simulink model "acrobot_sim_euler"  (R2013a)
settings: Solver=ode1  StartTime=0.0  StopTime=20  FixedStep=0.01  RelTol=1e-3
PreLoadFcn:
  | m1 = 1;
  | m2 = 1;
  | L1 = 1;
  | L2 = 1;
  | Lc1 = L1/2;
  | Lc2 = L2/2;
  | Ic1 = (Lc1*Lc1)/3;
  | Ic2 = (Lc2*Lc2)/3;
  | I1 = Ic1+m1*Lc1*Lc1;
  | I2 = Ic2+m2*Lc2*Lc2;
  | b1 = 0.4;
  | b2 = 0.4;
  | g = 9.8;
  | theta1_0 = -pi/8;
  | theta2_0 = 0;
StartFcn:
  | m1 = 1;
  | m2 = 1;
  | L1 = 1;
  | L2 = 1;
  | Lc1 = L1/2;
  | Lc2 = L2/2;
  | Ic1 = (Lc1*Lc1)/3;
  | Ic2 = (Lc2*Lc2)/3;
  | I1 = Ic1+m1*Lc1*Lc1;
  | I2 = Ic2+m2*Lc2*Lc2;
  | b1 = 0.4;
  | b2 = 0.4;
  | g = 9.8;
  | theta1_0 = -pi/8;
  | theta2_0 = 0;
libraries: mblibv1 x8, simulink x2
settings Model: Creator=Guy  LastModifiedBy=nightling
settings DataIOCC: SignalLoggingSaveFormat=ModelDataLogs
settings OptimizationCC: ExpressionDepthLimit=2147483647  InitFltsAndDblsToZero=on
settings DebuggingCC: AlgebraicLoopMsg=none  FcnCallInpInsideContextMsg=UseLocalSettings  StrictBusMsg=Warning
settings SFSimCC: SimParseCustomCode=off
settings GRTTargetCC: CombineOutputUpdateFcns=off  GRTInterface=on
settings SimMechanicsCC: VisOnUpdateDiagram=on  VisDuringSimulation=on  AutoFitVis=GROWTOFIT  LastVizWinPosition=[685 679 560 420]  CamPosition=[0.997125;-1.39973;13.4628;]  CamTarget=[0.997125;-1.39973;0;]  CamUpVector=[0;1;0;]  CamHeight=3.22959  VisBackgroundColor=[0.9;0.9;0.95;]  DefaultBodyColor=[1;0;0;]

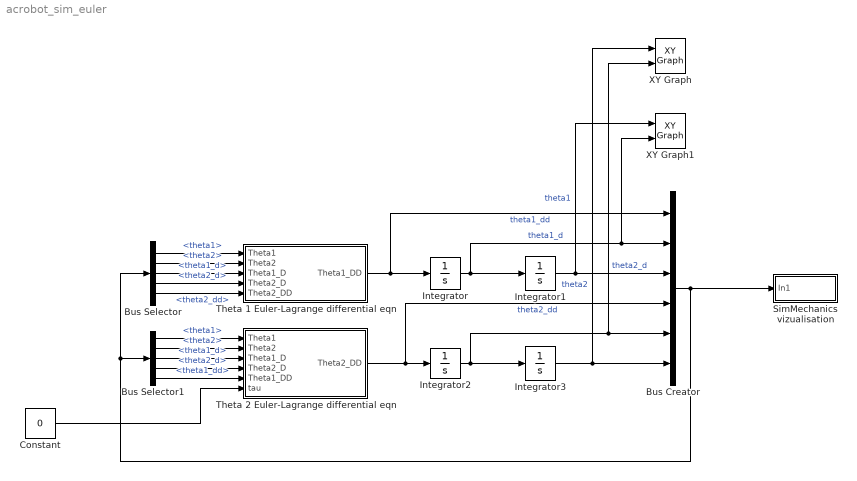
== system acrobot_sim_euler ==
  Bus Creator : BusCreator  Inputs=6
  Bus Selector : BusSelector  OutputSignals=theta1,theta2,theta1_d,theta2_d,theta2_dd
  Bus Selector1 : BusSelector  OutputSignals=theta1,theta2,theta1_d,theta2_d,theta1_dd
  Constant : Constant  Value=0
  Integrator : Integrator  InitialCondition=[0 ]
  Integrator1 : Integrator  InitialCondition=theta1_0
  Integrator2 : Integrator  InitialCondition="[0  ]"
  Integrator3 : Integrator  InitialCondition=theta2_0
  SimMechanics vizualisation : Subsystem
  Theta 1 Euler-Lagrange differential eqn : Subsystem
  Theta 2 Euler-Lagrange differential eqn : Subsystem
  XY Graph : simulink/Sinks/XY Graph  xmin=-0.5  xmax=0.5  ymin=-2  ymax=2  st=-1
  XY Graph1 : simulink/Sinks/XY Graph  xmin=-1  xmax=1  ymin=-5  ymax=5  st=-1
  wires:
  Integrator/1 -> XY Graph1/2, Bus Creator/2, Integrator1/1  "theta1_d"
  Integrator1/1 -> XY Graph1/1, Bus Creator/3  "theta1"
  Theta 1 Euler-Lagrange differential eqn/1(Theta1_DD) -> Bus Creator/1, Integrator/1  "theta1_dd"
  Theta 2 Euler-Lagrange differential eqn/1(Theta2_DD) -> Bus Creator/4, Integrator2/1  "theta2_dd"
  Integrator2/1 -> XY Graph/2, Bus Creator/5, Integrator3/1  "theta2_d"
  Integrator3/1 -> XY Graph/1, Bus Creator/6  "theta2"
  Bus Selector/1 -> Theta 1 Euler-Lagrange differential eqn/1(Theta1)  "<theta1>"
  Bus Selector/2 -> Theta 1 Euler-Lagrange differential eqn/2(Theta2)  "<theta2>"
  Bus Selector/5 -> Theta 1 Euler-Lagrange differential eqn/5(Theta2_DD)  "<theta2_dd>"
  Bus Selector/4 -> Theta 1 Euler-Lagrange differential eqn/4(Theta2_D)  "<theta2_d>"
  Bus Selector1/1 -> Theta 2 Euler-Lagrange differential eqn/1(Theta1)  "<theta1>"
  Bus Selector1/2 -> Theta 2 Euler-Lagrange differential eqn/2(Theta2)  "<theta2>"
  Bus Selector1/5 -> Theta 2 Euler-Lagrange differential eqn/5(Theta1_DD)  "<theta1_dd>"
  Bus Selector1/3 -> Theta 2 Euler-Lagrange differential eqn/3(Theta1_D)  "<theta1_d>"
  Bus Selector/3 -> Theta 1 Euler-Lagrange differential eqn/3(Theta1_D)  "<theta1_d>"
  Bus Selector1/4 -> Theta 2 Euler-Lagrange differential eqn/4(Theta2_D)  "<theta2_d>"
  Bus Creator/1 -> Bus Selector/1, Bus Selector1/1, SimMechanics vizualisation/1(In1)
  Constant/1 -> Theta 2 Euler-Lagrange differential eqn/6(tau)

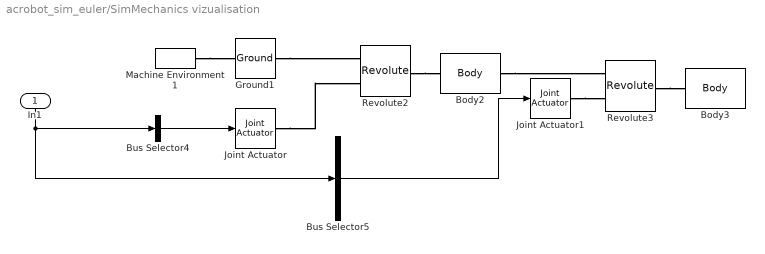
== system acrobot_sim_euler/SimMechanics vizualisation ==
  In1 : Inport
  Body2 : mblibv1/Bodies/Body  LConnTagsString=CS1  RConnTagsString=CS2  UpdateFromCAD=off  DialogClass=MechanicalBodyBlock  Mass=m1  MassUnits=kg  InertiaUnits=kg*m^2  Inertia=zeros(3)  Shape=Cylinder  ShapeDims=[1 1]  ShapeUnits=m  ShapeUse=false  Density=1  DensityUnits=kg/m^3  DensityUse=false  GraphicsMode=MACHINE_DEFAULT  BodyColorSelMode=COLORPALETTE  BodyColor=[0.043137 0.51765 0.78039]  AttachedToCS=CG  CG=Left$CG$[0 -L1/2 0]$CS1$CS1$m$[0 0 0]$Euler X-Y-Z$deg$WORLD$false$none  WorkingFrames=Left$CS1$[0 0 0]$Adjoining$Adjoining$m$[0 0 0]$Euler X-Y-Z$deg$WORLD$true$none#Right$CS2$[0 -L1 0]$CS1$CS1$m$[0 0 0]$Euler X-Y-Z$deg$WORLD$true$none  CGPos=[0 -L1/2 0]  CGRot=[0 0 0]  CS0Pos=[]  CS0Rot=[]  CS1Pos=[0 0 0]  CS1Rot=[0 0 0]  CS2Pos=[0 -L1 0]  CS2Rot=[0 0 0]  CS3Pos=[]  CS3Rot=[]  CS4Pos=[]  CS4Rot=[]  CS5Pos=[]  CS5Rot=[]  CS6Pos=[]  CS6Rot=[]  CS7Pos=[]  CS7Rot=[]  CS8Pos=[]  CS8Rot=[]  CS9Pos=[]  CS9Rot=[]  CS10Pos=[]  CS10Rot=[]  CS11Pos=[]  CS11Rot=[]  CS12Pos=[]  CS12Rot=[]  CS13Pos=[]  CS13Rot=[]  CS14Pos=[]  CS14Rot=[]  CS15Pos=[]  CS15Rot=[]  CS16Pos=[]  CS16Rot=[]  CS17Pos=[]  CS17Rot=[]  CS18Pos=[]  CS18Rot=[]  CS19Pos=[]  CS19Rot=[]  CS20Pos=[]  CS20Rot=[]
  Body3 : mblibv1/Bodies/Body  LConnTagsString=CS1  UpdateFromCAD=off  DialogClass=MechanicalBodyBlock  Mass=m2  MassUnits=kg  InertiaUnits=kg*m^2  Inertia=zeros(3)  Shape=Cylinder  ShapeDims=[1 1]  ShapeUnits=m  ShapeUse=false  Density=1  DensityUnits=kg/m^3  DensityUse=false  GraphicsMode=MACHINE_DEFAULT  BodyColorSelMode=COLORPALETTE  BodyColor=[0.043137 0.51765 0.78039]  AttachedToCS=CG  CG=Left$CG$[0 -L2/2 0]$CS1$CS1$m$[0 0 0]$Euler X-Y-Z$deg$WORLD$false$none  WorkingFrames=Left$CS1$[0 0 0]$Adjoining$Adjoining$m$[0 0 0]$Euler X-Y-Z$deg$WORLD$true$none#Right$CS2$[0 -L2 0]$CS1$CS1$m$[0 0 0]$Euler X-Y-Z$deg$WORLD$false$none  CGPos=[0 -L2/2 0]  CGRot=[0 0 0]  CS0Pos=[]  CS0Rot=[]  CS1Pos=[0 0 0]  CS1Rot=[0 0 0]  CS2Pos=[0 -L2 0]  CS2Rot=[0 0 0]  CS3Pos=[]  CS3Rot=[]  CS4Pos=[]  CS4Rot=[]  CS5Pos=[]  CS5Rot=[]  CS6Pos=[]  CS6Rot=[]  CS7Pos=[]  CS7Rot=[]  CS8Pos=[]  CS8Rot=[]  CS9Pos=[]  CS9Rot=[]  CS10Pos=[]  CS10Rot=[]  CS11Pos=[]  CS11Rot=[]  CS12Pos=[]  CS12Rot=[]  CS13Pos=[]  CS13Rot=[]  CS14Pos=[]  CS14Rot=[]  CS15Pos=[]  CS15Rot=[]  CS16Pos=[]  CS16Rot=[]  CS17Pos=[]  CS17Rot=[]  CS18Pos=[]  CS18Rot=[]  CS19Pos=[]  CS19Rot=[]  CS20Pos=[]  CS20Rot=[]
  Bus Selector4 : BusSelector  OutputSignals=theta1,theta1_d,theta1_dd  OutputAsBus=on
  Bus Selector5 : BusSelector  OutputSignals=theta2,theta2_d,theta2_dd  OutputAsBus=on
  Ground1 : mblibv1/Bodies/Ground  UpdateFromCAD=off  LeftPortType=env  RightPortType=workingframe  PhysicalDomain=Mechanical  DialogClass=GroundBlock  CoordPosition=[1 0 0]  CoordPositionUnits=m  StateVectorMgrId=1  MachineId=[2 0]  ShowEnvPort=on
  Joint Actuator : mblibv1/Sensors &  Actuators/Joint Actuator  UpdateFromCAD=off  PhysicalDomain=Mechanical  PortType=blob  ActuationStyle=Motion  AngleUnits=rad  ArcVelocityUnits=rad/s  ArcAccelerationUnits=rad/s^2  CoordPositionUnits=m  VelocityUnits=m/s  AccelerationUnits=m/s^2  ForceUnits=N  TorqueUnits=N*m  ActiveIO=on  Width=3  DialogClass=MechanicalActuatorBlock  Primitive=R1  ReferenceFrame=Absolute (World)
  Joint Actuator1 : mblibv1/Sensors &  Actuators/Joint Actuator  UpdateFromCAD=off  PhysicalDomain=Mechanical  PortType=blob  ActuationStyle=Motion  AngleUnits=rad  ArcVelocityUnits=rad/s  ArcAccelerationUnits=rad/s^2  CoordPositionUnits=m  VelocityUnits=m/s  AccelerationUnits=m/s^2  ForceUnits=N  TorqueUnits=N*m  ActiveIO=on  Width=3  DialogClass=MechanicalActuatorBlock  Primitive=R1  ReferenceFrame=Absolute (World)
  Machine Environment1 : mblibv1/Bodies/Machine Environment  PortType=env  PhysicalDomain=Mechanical  DialogTemplateClass=MECH.MachineEnvironment  SyncWhenCopied=off  Gravity=[0 -9.81 0]  GravityUnits=m/s^2  GravityAsSignal=off  Dimensionality=Auto-detect  AnalysisType=Forward dynamics  LinearAssemblyTolerance=1e-3  LinearAssemblyToleranceUnits=m  AngularAssemblyTolerance=1e-3  AngularAssemblyToleranceUnits=rad  ConstraintSolverType=Stabilizing  ConstraintRelTolerance=1e-4  ConstraintAbsTolerance=1e-4  UseRobustSingularityHandling=off  RedundancyAnalysisToleranceType=Automatically select tolerance  RedundancyAnalysisTolerance=1e-14  StatePerturbationType=Fixed  PerturbationSize=1e-5  VisualizeMachine=on  BodyVisualizationType=Use model default body geometries  BodyColorSelMode=Use model default  DefaultBodyColor=[1 0 0]
  Revolute2 : mblibv1/Joints/Revolute  LConnTagsString=__newl0|SA1  RConnTagsString=__newr0  UpdateFromCAD=off  NumSAPorts=1  CutJoint=off  MarkAsCut=off  Primitives=prismatic  PrimitiveProps=R1$World$[0 0 1]$revolute  DialogClass=JointBlock  R1Axis=[0 0 1]
  Revolute3 : mblibv1/Joints/Revolute  LConnTagsString=__newl0|SA1  RConnTagsString=__newr0  UpdateFromCAD=off  NumSAPorts=1  CutJoint=off  MarkAsCut=off  Primitives=prismatic  PrimitiveProps=R1$World$[0 0 1]$revolute  DialogClass=JointBlock  R1Axis=[0 0 1]
  wires:
  Bus Selector4/1 -> Joint Actuator/1
  In1/1 -> Bus Selector5/1, Bus Selector4/1
  Bus Selector5/1 -> Joint Actuator1/1
  connections:
  Revolute2/RConn1 -- Body2/LConn1
  Body2/RConn1 -- Revolute3/LConn1
  Revolute3/RConn1 -- Body3/LConn1
  Machine Environment1/RConn1 -- Ground1/LConn1
  Ground1/RConn1 -- Revolute2/LConn1
  Joint Actuator/RConn1 -- Revolute2/LConn2
  Joint Actuator1/RConn1 -- Revolute3/LConn2

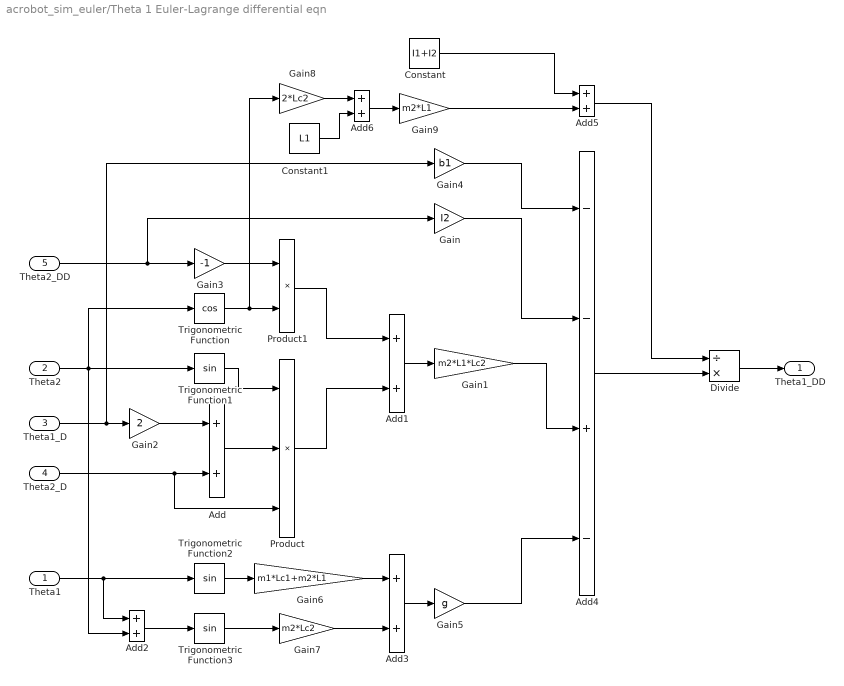
== system acrobot_sim_euler/Theta 1 Euler-Lagrange differential eqn ==
  Theta1 : Inport
  Theta2 : Inport  Port=2
  Theta1_D : Inport  Port=3
  Theta2_D : Inport  Port=4
  Theta2_DD : Inport  Port=5
  Add{,1..3,5..6} (6 alike) : Sum
  Add4 : Sum  Inputs=--+-
  Constant : Constant  Value=I1+I2
  Constant1 : Constant  Value=L1
  Divide : Product  Inputs=/*
  Gain : Gain  Gain=I2
  Gain1 : Gain  Gain=m2*L1*Lc2
  Gain2 : Gain  Gain=2
  Gain3 : Gain  Gain=-1
  Gain4 : Gain  Gain=b1
  Gain5 : Gain  Gain=g
  Gain6 : Gain  Gain=m1*Lc1+m2*L1
  Gain7 : Gain  Gain=m2*Lc2
  Gain8 : Gain  Gain=2*Lc2
  Gain9 : Gain  Gain=m2*L1
  Product : Product  Inputs=3
  Product1 : Product
  Trigonometric Function : Trigonometry  Operator=cos
  Trigonometric Function1 : Trigonometry
  Trigonometric Function2 : Trigonometry
  Trigonometric Function3 : Trigonometry
  Theta1_DD : Outport
  wires:
  Theta2/1 -> Add2/2, Trigonometric Function/1, Trigonometric Function1/1
  Theta2_D/1 -> Product/3, Add/2
  Gain2/1 -> Add/1
  Theta1_D/1 -> Gain4/1, Gain2/1
  Add/1 -> Product/2
  Trigonometric Function1/1 -> Product/1
  Theta2_DD/1 -> Gain/1, Gain3/1
  Gain3/1 -> Product1/1
  Trigonometric Function/1 -> Product1/2, Gain8/1
  Product1/1 -> Add1/1
  Product/1 -> Add1/2
  Add1/1 -> Gain1/1
  Theta1/1 -> Add2/1, Trigonometric Function2/1
  Trigonometric Function2/1 -> Gain6/1
  Add2/1 -> Trigonometric Function3/1
  Trigonometric Function3/1 -> Gain7/1
  Gain6/1 -> Add3/1
  Gain7/1 -> Add3/2
  Add3/1 -> Gain5/1
  Gain4/1 -> Add4/1
  Gain/1 -> Add4/2
  Gain1/1 -> Add4/3
  Gain5/1 -> Add4/4
  Gain9/1 -> Add5/2
  Constant/1 -> Add5/1
  Add4/1 -> Divide/2
  Add5/1 -> Divide/1
  Divide/1 -> Theta1_DD/1
  Gain8/1 -> Add6/1
  Constant1/1 -> Add6/2
  Add6/1 -> Gain9/1

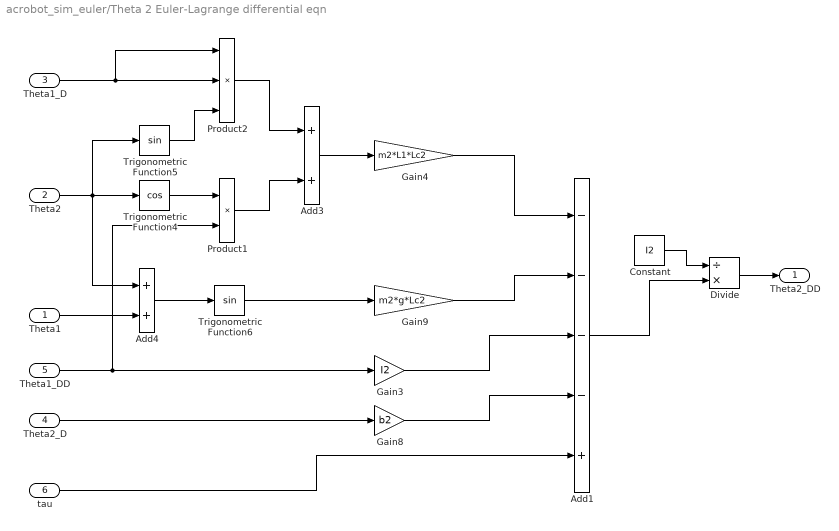
== system acrobot_sim_euler/Theta 2 Euler-Lagrange differential eqn ==
  Theta1 : Inport
  Theta2 : Inport  Port=2
  Theta1_D : Inport  Port=3
  Theta2_D : Inport  Port=4
  Theta1_DD : Inport  Port=5
  tau : Inport  Port=6
  Add1 : Sum  Inputs=----+
  Add3 : Sum
  Add4 : Sum
  Constant : Constant  Value=I2
  Divide : Product  Inputs=/*
  Gain3 : Gain  Gain=I2
  Gain4 : Gain  Gain=m2*L1*Lc2
  Gain8 : Gain  Gain=b2
  Gain9 : Gain  Gain=m2*g*Lc2
  Product1 : Product
  Product2 : Product  Inputs=3
  Trigonometric Function4 : Trigonometry  Operator=cos
  Trigonometric Function5 : Trigonometry
  Trigonometric Function6 : Trigonometry
  Theta2_DD : Outport
  wires:
  Theta2/1 -> Add4/1, Trigonometric Function5/1, Trigonometric Function4/1
  Divide/1 -> Theta2_DD/1
  Theta1_DD/1 -> Product1/2, Gain3/1
  Trigonometric Function4/1 -> Product1/1
  Theta1_D/1 -> Product2/1, Product2/2
  Trigonometric Function5/1 -> Product2/3
  Product2/1 -> Add3/1
  Product1/1 -> Add3/2
  Add3/1 -> Gain4/1
  Theta2_D/1 -> Gain8/1
  Theta1/1 -> Add4/2
  Add4/1 -> Trigonometric Function6/1
  Trigonometric Function6/1 -> Gain9/1
  Gain4/1 -> Add1/1
  Gain9/1 -> Add1/2
  Gain3/1 -> Add1/3
  Gain8/1 -> Add1/4
  tau/1 -> Add1/5
  Add1/1 -> Divide/2
  Constant/1 -> Divide/1
